simulink model "Demo_3D_FlexRoads_cs"  (R2014b)
settings: Solver=ode5  SolverMode=SingleTasking  StartTime=0.0  StopTime=107  FixedStep=1/200  RelTol=1e-3
PreLoadFcn:
  | mbxruntime.callbacks.PreLoadFcn(bdroot);
  | check_NUTS_defined;
  | 
  | assignin('base',['model_closed_' bdroot],false);
PostLoadFcn:
  | mbxruntime.callbacks.PostLoadFcn(bdroot);
InitFcn:
  | mbxruntime.callbacks.InitFcn(bdroot);
StartFcn:
  | mbxruntime.callbacks.StartFcn(bdroot);
StopFcn:
  | mbxruntime.callbacks.StopFcn(bdroot);
model workspace: external: MAT-File .\Demo_3D_FlexRoads_cs_hws.mat (data not in the file)
undefined symbols (not defined in the file or in its folder): InitImageOutputDir, warningInitialVelocity, x0
undefined symbols (not defined in the file): Demo_3D_FlexRoads_cs_51f4b8db1f5c5ce4, Demo_3D_FlexRoads_cs_6db096e0daa372af, Demo_3D_FlexRoads_cs_Audi_A8_1_Dynamics_Simple_3D_initialPitch, Demo_3D_FlexRoads_cs_Audi_A8_1_Dynamics_Simple_3D_initialRoll, Demo_3D_FlexRoads_cs_Audi_A8_1_Dynamics_Simple_3D_initialX, Demo_3D_FlexRoads_cs_Audi_A8_1_Dynamics_Simple_3D_initialY, Demo_3D_FlexRoads_cs_Audi_A8_1_Dynamics_Simple_3D_initialYaw, Demo_3D_FlexRoads_cs_Audi_A8_1_Dynamics_Simple_3D_initialZ, Demo_3D_FlexRoads_cs_Audi_A8_1_PreScan_Contact_Sensor_Pitch0, Demo_3D_FlexRoads_cs_Audi_A8_1_PreScan_Contact_Sensor_Roll0, Demo_3D_FlexRoads_cs_Audi_A8_1_PreScan_Contact_Sensor_x0, Demo_3D_FlexRoads_cs_Audi_A8_1_PreScan_Contact_Sensor_y0, Demo_3D_FlexRoads_cs_Audi_A8_1_PreScan_Contact_Sensor_Yaw0, Demo_3D_FlexRoads_cs_Audi_A8_1_PreScan_Contact_Sensor_z0, Demo_3D_FlexRoads_cs_Ford_FocusWagon_1_Path_pathUniqueID, WheelL0, WheelL1, WheelR0, WheelR1
libraries: simulink x34, simulink_extras x10, PreScanSimulinkLibrary x7
(part 5 of 6)

== system Demo_3D_FlexRoads_cs/Audi_A8_1/PreScan_Contact_Sensor/Wheels Local to World/conv_TransWheelFR ==
  transISO [m] : Inport
  Gain1 : Gain  Gain=Gain_xISO
  Gain2 : Gain  Gain=Gain_yISO
  Gain3 : Gain  Gain=Gain_zISO
  Mux2 : Mux  Inputs=3
  Sum : Sum  Inputs=|++
  pos_ini_Visu : Subsystem
  transISO2Visu : Subsystem
  transVisu [m] : Outport
  wires:
  Gain3/1 -> Mux2/3
  Gain2/1 -> Mux2/2
  Gain1/1 -> Mux2/1
  Sum/1 -> transVisu [m]/1
  pos_ini_Visu/1(pos_ini_Visu) -> Sum/2
  Mux2/1 -> Sum/1
  transISO [m]/1 -> transISO2Visu/1(transISO)
  transISO2Visu/1(trans_x_Visu) -> Gain1/1
  transISO2Visu/2(trans_y_Visu) -> Gain2/1
  transISO2Visu/3(trans_z_Visu) -> Gain3/1

== system Demo_3D_FlexRoads_cs/Audi_A8_1/PreScan_Contact_Sensor/Wheels Local to World/conv_TransWheelRL ==
  transISO [m] : Inport
  Gain1 : Gain  Gain=Gain_xISO
  Gain2 : Gain  Gain=Gain_yISO
  Gain3 : Gain  Gain=Gain_zISO
  Mux2 : Mux  Inputs=3
  Sum : Sum  Inputs=|++
  pos_ini_Visu : Subsystem
  transISO2Visu : Subsystem
  transVisu [m] : Outport
  wires:
  Gain3/1 -> Mux2/3
  Gain2/1 -> Mux2/2
  Gain1/1 -> Mux2/1
  Sum/1 -> transVisu [m]/1
  pos_ini_Visu/1(pos_ini_Visu) -> Sum/2
  Mux2/1 -> Sum/1
  transISO2Visu/3(trans_z_Visu) -> Gain3/1
  transISO2Visu/2(trans_y_Visu) -> Gain2/1
  transISO [m]/1 -> transISO2Visu/1(transISO)
  transISO2Visu/1(trans_x_Visu) -> Gain1/1

== system Demo_3D_FlexRoads_cs/Audi_A8_1/PreScan_Contact_Sensor/Wheels Local to World/conv_TransWheelRR ==
  transISO [m] : Inport
  Gain1 : Gain  Gain=Gain_xISO
  Gain2 : Gain  Gain=Gain_yISO
  Gain3 : Gain  Gain=Gain_zISO
  Mux2 : Mux  Inputs=3
  Sum : Sum  Inputs=|++
  pos_ini_Visu : Subsystem
  transISO2Visu : Subsystem
  transVisu [m] : Outport
  wires:
  Gain3/1 -> Mux2/3
  Gain2/1 -> Mux2/2
  Gain1/1 -> Mux2/1
  Sum/1 -> transVisu [m]/1
  pos_ini_Visu/1(pos_ini_Visu) -> Sum/2
  Mux2/1 -> Sum/1
  transISO2Visu/3(trans_z_Visu) -> Gain3/1
  transISO2Visu/2(trans_y_Visu) -> Gain2/1
  transISO [m]/1 -> transISO2Visu/1(transISO)
  transISO2Visu/1(trans_x_Visu) -> Gain1/1

== system Demo_3D_FlexRoads_cs/Audi_A8_1/SELF_Demux/compas converter/cart2compas ==
  Angle [deg] : Inport
  Constant : Constant  Value=90
  Constant1 : Constant  Value=360
  Gain : Gain  Gain=1/360
  Gain1 : Gain  Gain=360
  Gain2 : Gain  Gain=-1
  Rounding Function : Rounding
  Sum : Sum  Inputs=|-+
  Sum1 : Sum  Inputs=-+|
  Sum2 : Sum  Inputs=++|
  heading [deg] : Outport
  wires:
  Gain/1 -> Rounding Function/1
  Rounding Function/1 -> Gain1/1
  Gain1/1 -> Sum/1
  Angle [deg]/1 -> Sum1/2
  Sum/1 -> Gain2/1
  Sum1/1 -> Gain/1, Sum/2
  Constant/1 -> Sum1/1
  Gain2/1 -> Sum2/2
  Constant1/1 -> Sum2/1
  Sum2/1 -> heading [deg]/1

== system Demo_3D_FlexRoads_cs/Ford_FocusWagon_1/SELF_Demux/compas converter/cart2compas ==
  Angle [deg] : Inport
  Constant : Constant  Value=90
  Constant1 : Constant  Value=360
  Gain : Gain  Gain=1/360
  Gain1 : Gain  Gain=360
  Gain2 : Gain  Gain=-1
  Rounding Function : Rounding
  Sum : Sum  Inputs=|-+
  Sum1 : Sum  Inputs=-+|
  Sum2 : Sum  Inputs=++|
  heading [deg] : Outport
  wires:
  Gain/1 -> Rounding Function/1
  Rounding Function/1 -> Gain1/1
  Gain1/1 -> Sum/1
  Angle [deg]/1 -> Sum1/2
  Sum/1 -> Gain2/1
  Sum1/1 -> Gain/1, Sum/2
  Constant/1 -> Sum1/1
  Gain2/1 -> Sum2/2
  Constant1/1 -> Sum2/1
  Sum2/1 -> heading [deg]/1

== system Demo_3D_FlexRoads_cs/Audi_A8_1/Dynamics_Simple_3D/Chassis/Bicycle_model_[XYZ]/Fyi --> Fy // Mz ==
  DeltaWheel_[rad] : Inport
  Fy_f_[N] : Inport  Port=2
  Fy_r_[N] : Inport  Port=3
  Fy : Fcn  Expr=u(2)*cos(u(1)) + u(3)
  Mux1 : Mux  Inputs=3
  Mz : Fcn  Expr=u(2)*p.a*cos(u(1)) - u(3)*p.b
  Fy_[N] : Outport  InitialOutput=0
  Mz_[Nm] : Outport  Port=2  InitialOutput=0
  wires:
  DeltaWheel_[rad]/1 -> Mux1/1  "DeltaWheel_[rad]"
  Mz/1 -> Mz_[Nm]/1
  Fy/1 -> Fy_[N]/1
  Mux1/1 -> Mz/1, Fy/1
  Fy_f_[N]/1 -> Mux1/2
  Fy_r_[N]/1 -> Mux1/3

== system Demo_3D_FlexRoads_cs/Audi_A8_1/Dynamics_Simple_3D/Chassis/Bicycle_model_[XYZ]/RoadContact ==
  TyreInfo_in : Inport
  Penetration depth : Subsystem
  RoadGeometry : Subsystem
  depth_FL [m] : Outport
  depth_FR [m] : Outport  Port=2
  depth_RL [m] : Outport  Port=3
  depth_RR [m] : Outport  Port=4
  z : Outport  Port=5
  slope : Outport  Port=6
  banking : Outport  Port=7
  wires:
  Penetration depth/4(depth_RR [m]) -> depth_RR [m]/1
  Penetration depth/3(depth_RL [m]) -> depth_RL [m]/1
  Penetration depth/2(depth_FR [m]) -> depth_FR [m]/1
  Penetration depth/1(depth_FL [m]) -> depth_FL [m]/1
  TyreInfo_in/1 -> Penetration depth/1(TyreInfo_in), RoadGeometry/1(TyreInfo_in)
  RoadGeometry/1(z) -> z/1
  RoadGeometry/2(slope) -> slope/1
  RoadGeometry/3(banking) -> banking/1

== system Demo_3D_FlexRoads_cs/Audi_A8_1/Dynamics_Simple_3D/Chassis/Bicycle_model_[XYZ]/X_Motion ==
  DriveTorque_[Nm] : Inport
  BrakePressure_[bar] : Inport  Port=2
  v0_[ms-1] : Inport  Port=3
  slope_[rad] : Inport  Port=4
  vy_[ms-1] : Inport  Port=5
  dYaw_[rads-1] : Inport  Port=6
  Air&RoadResistance : Subsystem
  BrakeSystem : Subsystem
  Configurable Subsystem : Subsystem  BlockChoice=Discrete-Time Integrator  mask{ComputationMode=ComputationMode}
      mask prompts: ComputationMode "Computation mode:"
      mask init:
      | SetComputationMode(gcb,ComputationMode);
      settings: AttributesFormatString=%<BlockChoice>  OpenFcn=BringToFront(gcb);  MemberBlocks=Discrete-Time Integrator,Integrator
      settings: TemplateBlock=|
      | PreScanSimulinkLibrary/Configurable Subsystems/integral with reset and initial condition/Configurable
      | Subsystem
  Configurable Subsystem1 : Subsystem  BlockChoice=Discrete Torsional damping  mask{ComputationMode=ComputationMode}
      mask prompts: ComputationMode "Compuation mode:"
      mask init:
      | SetComputationMode(gcb,ComputationMode);
      settings: AttributesFormatString=%<BlockChoice>  OpenFcn=BringToFront(gcb);  MemberBlocks=Discrete Torsional damping,Torsional damping
      settings: TemplateBlock=|
      | PreScanSimulinkLibrary/Configurable Subsystems/TransferFunction
      | Torsional damping/Configurable
      | Subsystem
  Divide : Product  Inputs=**
  Gain : Gain  Gain=1/p.Rw
  Gain1 : Gain  Gain=p.Rw
  Max RPM and zero- velocity detection : Subsystem
  No contact rear wheels : Subsystem
  No contact wheels : Subsystem
  Slope Force : Subsystem
  Sum : Sum  Inputs=+-  SaturateOnIntegerOverflow=on  InputSameDT=on  OutDataTypeStr=Inherit: Same as first input
  Sum1 : Sum  SaturateOnIntegerOverflow=on  InputSameDT=on  OutDataTypeStr=Inherit: Same as first input
  Sum2 : Sum  Inputs=++-  SaturateOnIntegerOverflow=on  InputSameDT=on  OutDataTypeStr=Inherit: Same as first input
  inertia : Gain  Gain=1/p.m  SaturateOnIntegerOverflow=on  OutDataTypeStr=Inherit: Same as input  ParamDataTypeStr=Inherit: Same as input
  vx_[ms-1] : Outport
  ax_[ms-2] : Outport  Port=2
  wires:
  No contact rear wheels/1(ForceOut [N]) -> Sum/1
  Sum/1 -> Sum2/1  "sumForce_[N]"
  No contact wheels/1(ForceOut [N]) -> Sum2/3
  BrakeSystem/1(BrakeForce) -> No contact wheels/1(ForceIn [N])
  [slopeT] -> Max RPM and zero- velocity detection/3(Slope Torque)
  slope_[rad]/1 -> Slope Force/1(slope_[rad]), Air&RoadResistance/2(slope_[rad])
  Gain1/1 -> [slopeT]
  Slope Force/1(SlopeForce_[N]) -> Gain1/1, Sum2/2
  Gain/1 -> No contact rear wheels/1(ForceIn [N])
  Divide/1 -> Sum1/1
  dYaw_[rads-1]/1 -> Divide/2
  vy_[ms-1]/1 -> Divide/1
  BrakeSystem/2(BrakeTorqueAbs) -> [BT]
  [BT] -> Max RPM and zero- velocity detection/4(Brake Torque)
  [DT] -> Max RPM and zero- velocity detection/2(Drive Torque)
  v0_[ms-1]/1 -> Max RPM and zero- velocity detection/5(v0)
  Max RPM and zero- velocity detection/3(x0) -> Configurable Subsystem/3(In3)
  Max RPM and zero- velocity detection/2(vx_reset) -> Configurable Subsystem/2(In2)
  Max RPM and zero- velocity detection/1(ax_out) -> ax_[ms-2]/1, Configurable Subsystem/1(In1)  "ax [ms-2]"
  Configurable Subsystem1/1(Out1) -> Gain/1, [DT]
  Sum1/1 -> Max RPM and zero- velocity detection/1(ax)
  DriveTorque_[Nm]/1 -> Configurable Subsystem1/1(In1)  "DriveTorque_[Nm]"
  BrakePressure_[bar]/1 -> BrakeSystem/2(BrakePressure_[bar])  "BrakePressure_[bar]"
  Configurable Subsystem/1(Out1) -> Max RPM and zero- velocity detection/6(vx), BrakeSystem/1(vx_[ms-1]), Air&RoadResistance/1(vx_[ms-1]), vx_[ms-1]/1  "vx_[ms-1]"
  Air&RoadResistance/1(Resistance_Force) -> Sum/2
  Sum2/1 -> inertia/1
  inertia/1 -> Sum1/2  "dw[rads-2]"

== system Demo_3D_FlexRoads_cs/Audi_A8_1/Dynamics_Simple_3D/Chassis/Bicycle_model_[XYZ]/Y & Yaw_Motion ==
  |vx|_[ms-1] : Inport
  Fy_[N] : Inport  Port=2
  Mz_[Nm] : Inport  Port=3
  Compare To Zero : simulink/Logic and Bit Operations/Compare To Zero  relop===  OutDataTypeStr=boolean  ZeroCross=off
  Configurable Subsystem : Subsystem  BlockChoice=Discrete-Time Integrator  mask{ComputationMode=ComputationMode}
      mask prompts: ComputationMode "Computation mode:"
      mask init:
      | SetComputationMode(gcb,ComputationMode);
      settings: AttributesFormatString=%<BlockChoice>  OpenFcn=BringToFront(gcb);  MemberBlocks=Discrete-Time Integrator,Integrator
      settings: TemplateBlock=|
      | PreScanSimulinkLibrary/Configurable Subsystems/integral with reset/Configurable
      | Subsystem
  Configurable Subsystem1 : Subsystem  BlockChoice=Discrete-Time Integrator  mask{ComputationMode=ComputationMode}
      mask prompts: ComputationMode "Computation mode:"
      mask init:
      | SetComputationMode(gcb,ComputationMode);
      settings: AttributesFormatString=%<BlockChoice>  OpenFcn=BringToFront(gcb);  MemberBlocks=Discrete-Time Integrator,Integrator
      settings: TemplateBlock=|
      | PreScanSimulinkLibrary/Configurable Subsystems/integral with reset/Configurable
      | Subsystem
  Configurable Subsystem2 : Subsystem  BlockChoice=Discrete-Time Integrator  mask{ComputationMode=ComputationMode}
      link override Discrete-Time Integrator: IntegratorMethod=Integration: Backward Euler
      mask prompts: ComputationMode "Computation mode:"
      mask init:
      | SetComputationMode(gcb,ComputationMode);
      settings: AttributesFormatString=%<BlockChoice>  OpenFcn=BringToFront(gcb);  MemberBlocks=Discrete-Time Integrator,Integrator
      settings: TemplateBlock=|
      | PreScanSimulinkLibrary/Configurable Subsystems/integral/Configurable
      | Subsystem1
  Fcn1 : Fcn  Expr=u(1)*u(3)
  Gain : Gain  Gain=1/p.m  SaturateOnIntegerOverflow=on  OutDataTypeStr=Inherit: Same as input  ParamDataTypeStr=Inherit: Same as input
  Gain1 : Gain  Gain=1/p.J_zz  SaturateOnIntegerOverflow=on  OutDataTypeStr=Inherit: Same as input  ParamDataTypeStr=Inherit: Same as input
  Sum1 : Sum  Inputs=-+  SaturateOnIntegerOverflow=on  InputSameDT=on  OutDataTypeStr=Inherit: Same as first input
  mux : Mux  Inputs=3
  |vx|_[ms-1]1 : Outport  InitialOutput=0
  vy_[ms-1] : Outport  Port=2  InitialOutput=0
  ay_[ms-2] : Outport  Port=3  InitialOutput=0
  dYawAngle_[rads-1] : Outport  Port=4  InitialOutput=0
  YawAngle_[rad] : Outport  Port=5  InitialOutput=0
  wires:
  Configurable Subsystem1/1(Out1) -> mux/3, dYawAngle_[rads-1]/1, Configurable Subsystem2/1(In1)  "dYawAngle_[rads-1]"
  Configurable Subsystem/1(Out1) -> mux/2, vy_[ms-1]/1  "vy_[ms-1]"
  |vx|_[ms-1]/1 -> mux/1, |vx|_[ms-1]1/1, Compare To Zero/1  "|vx|_[ms-1]"
  mux/1 -> Fcn1/1  "|vx|_[ms-1]_vy_[ms-1]_dYawAngle_[rads-1]"
  Fcn1/1 -> Sum1/1  "|vx|*dYawAngle_[ms-2]"
  Sum1/1 -> Configurable Subsystem/1(In1)  "dvy_[ms-2]"
  Fy_[N]/1 -> Gain/1  "Fy_[N]"
  Mz_[Nm]/1 -> Gain1/1  "Mz_[Nm]"
  Configurable Subsystem2/1(Out1) -> YawAngle_[rad]/1
  Compare To Zero/1 -> [reset]
  [reset] -> Configurable Subsystem1/2(In2)
  [reset] -> Configurable Subsystem/2(In2)
  Gain/1 -> ay_[ms-2]/1, Sum1/2  "ddy_[ms-2]"
  Gain1/1 -> Configurable Subsystem1/1(In1)  "ddYawAngle_[rads-2]"

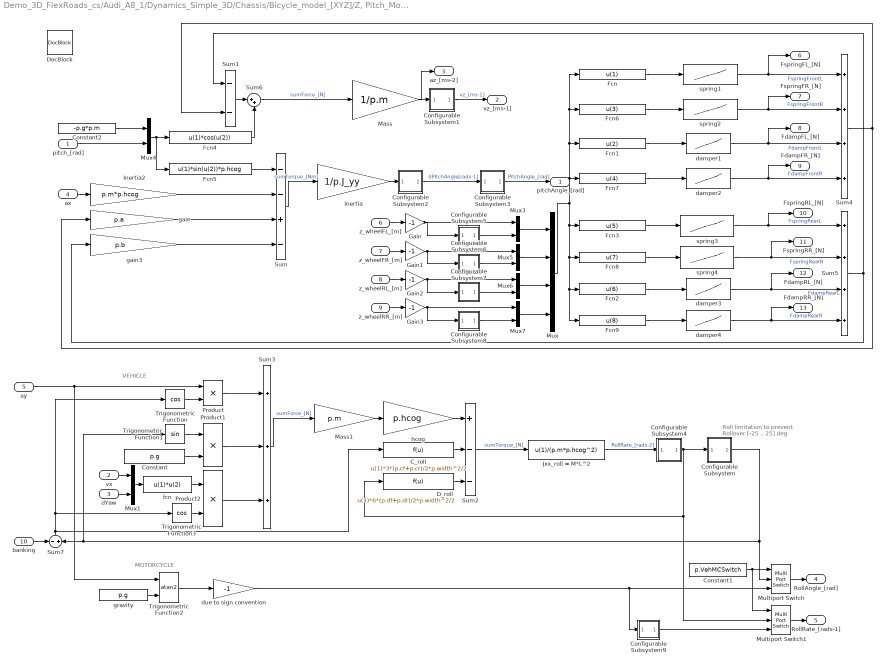
== system Demo_3D_FlexRoads_cs/Audi_A8_1/Dynamics_Simple_3D/Chassis/Bicycle_model_[XYZ]/Z, Pitch_Motion & Roll_Motion ==
  note: MOTORCYCLE
  note: Roll limitation
      | to prevent
      | Rollover
      | [-25 .. 25] deg
  note: VEHICLE
  pitch_[rad] : Inport
  vx : Inport  Port=2
  dYaw : Inport  Port=3
  ax : Inport  Port=4
  ay : Inport  Port=5
  z_wheelFL_[m] : Inport  Port=6
  z_wheelFR_[m] : Inport  Port=7
  z_wheelRL_[m] : Inport  Port=8
  z_wheelRR_[m] : Inport  Port=9
  banking : Inport  Port=10
  C_roll : Fcn  Expr=u(1)*3*(p.cf+p.cr)/2*p.width^2/2
  Configurable Subsystem : Subsystem  BlockChoice=Discrete-Time Integrator  mask{ComputationMode=ComputationMode}
      mask prompts: ComputationMode "Computation mode:"
      mask init:
      | SetComputationMode(gcb,ComputationMode);
      settings: AttributesFormatString=%<BlockChoice>  OpenFcn=BringToFront(gcb);  MemberBlocks=Discrete-Time Integrator,Integrator
      settings: TemplateBlock=|
      | PreScanSimulinkLibrary/Configurable Subsystems/integral with limits
      | for roll motion/Configurable
      | Subsystem
  Configurable Subsystem1 : Subsystem  BlockChoice=Discrete-Time Integrator  mask{ComputationMode=ComputationMode}
      mask prompts: ComputationMode "Computation mode:"
      mask init:
      | SetComputationMode(gcb,ComputationMode);
      settings: AttributesFormatString=%<BlockChoice>  OpenFcn=BringToFront(gcb);  MemberBlocks=Discrete-Time Integrator,Integrator
      settings: TemplateBlock=|
      | PreScanSimulinkLibrary/Configurable Subsystems/integral/Configurable
      | Subsystem1
  Configurable Subsystem2 : Subsystem  BlockChoice=Discrete-Time Integrator  mask{ComputationMode=ComputationMode}
      mask prompts: ComputationMode "Computation mode:"
      mask init:
      | SetComputationMode(gcb,ComputationMode);
      settings: AttributesFormatString=%<BlockChoice>  OpenFcn=BringToFront(gcb);  MemberBlocks=Discrete-Time Integrator,Integrator
      settings: TemplateBlock=|
      | PreScanSimulinkLibrary/Configurable Subsystems/integral/Configurable
      | Subsystem1
  Configurable Subsystem3 : Subsystem  BlockChoice=Discrete-Time Integrator  mask{ComputationMode=ComputationMode}
      mask prompts: ComputationMode "Computation mode:"
      mask init:
      | SetComputationMode(gcb,ComputationMode);
      settings: AttributesFormatString=%<BlockChoice>  OpenFcn=BringToFront(gcb);  MemberBlocks=Discrete-Time Integrator,Integrator
      settings: TemplateBlock=|
      | PreScanSimulinkLibrary/Configurable Subsystems/integral/Configurable
      | Subsystem1
  Configurable Subsystem4 : Subsystem  BlockChoice=Discrete-Time Integrator  mask{ComputationMode=ComputationMode}
      mask prompts: ComputationMode "Computation mode:"
      mask init:
      | SetComputationMode(gcb,ComputationMode);
      settings: AttributesFormatString=%<BlockChoice>  OpenFcn=BringToFront(gcb);  MemberBlocks=Discrete-Time Integrator,Integrator
      settings: TemplateBlock=|
      | PreScanSimulinkLibrary/Configurable Subsystems/integral/Configurable
      | Subsystem1
  Configurable Subsystem5 : Subsystem  BlockChoice=Discrete Derivative  mask{ComputationMode=ComputationMode}
      mask prompts: ComputationMode "Computation mode:"
      mask init:
      | SetComputationMode(gcb,ComputationMode);
      settings: AttributesFormatString=%<BlockChoice>  OpenFcn=BringToFront(gcb);  MemberBlocks=Derivative,Discrete Derivative
      settings: TemplateBlock=|
      | PreScanSimulinkLibrary/Configurable Subsystems/Derivative/Configurable
      | Subsystem
  Configurable Subsystem6 : Subsystem  BlockChoice=Discrete Derivative  mask{ComputationMode=ComputationMode}
      mask prompts: ComputationMode "Computation mode:"
      mask init:
      | SetComputationMode(gcb,ComputationMode);
      settings: AttributesFormatString=%<BlockChoice>  OpenFcn=BringToFront(gcb);  MemberBlocks=Derivative,Discrete Derivative
      settings: TemplateBlock=|
      | PreScanSimulinkLibrary/Configurable Subsystems/Derivative/Configurable
      | Subsystem
  Configurable Subsystem7 : Subsystem  BlockChoice=Discrete Derivative  mask{ComputationMode=ComputationMode}
      mask prompts: ComputationMode "Computation mode:"
      mask init:
      | SetComputationMode(gcb,ComputationMode);
      settings: AttributesFormatString=%<BlockChoice>  OpenFcn=BringToFront(gcb);  MemberBlocks=Derivative,Discrete Derivative
      settings: TemplateBlock=|
      | PreScanSimulinkLibrary/Configurable Subsystems/Derivative/Configurable
      | Subsystem
  Configurable Subsystem8 : Subsystem  BlockChoice=Discrete Derivative  mask{ComputationMode=ComputationMode}
      mask prompts: ComputationMode "Computation mode:"
      mask init:
      | SetComputationMode(gcb,ComputationMode);
      settings: AttributesFormatString=%<BlockChoice>  OpenFcn=BringToFront(gcb);  MemberBlocks=Derivative,Discrete Derivative
      settings: TemplateBlock=|
      | PreScanSimulinkLibrary/Configurable Subsystems/Derivative/Configurable
      | Subsystem
  Configurable Subsystem9 : Subsystem  BlockChoice=Discrete Derivative  mask{ComputationMode=ComputationMode}
      mask prompts: ComputationMode "Computation mode:"
      mask init:
      | SetComputationMode(gcb,ComputationMode);
      settings: AttributesFormatString=%<BlockChoice>  OpenFcn=BringToFront(gcb);  MemberBlocks=Derivative,Discrete Derivative
      settings: TemplateBlock=|
      | PreScanSimulinkLibrary/Configurable Subsystems/Derivative/Configurable
      | Subsystem
  Constant : Constant  Value=p.g
  Constant1 : Constant  Value=p.VehMCSwitch
  Constant2 : Constant  Value=-p.g*p.m
  D_roll : Fcn  Expr=u(1)*6*(p.df+p.dr)/2*p.width^2/2
  DocBlock : simulink/Model-Wide Utilities/DocBlock  DocumentType=Text
      content=|
      | This block determines the vertical, pitch and roll motions.
      |
      | The z motion is calculated by summing up all the forces that act in the
      | direction normal to the road:
      | - forces exerted by the suspensions (spring and dampers);
      | - vertical component of the force that is generated by the
      |   gravitational acceleration;
      | and then diving by the vehicle mass.
      |
      | The pitch motion is calculated by summing up all the torques that act
      | around the y-axis of the vehicle:
      | - forces exerted by the suspensions (spring and dampers);
      | - force generated by the longitudinal acceleration of the vehicle;
      | - longitudinal component of the force that is generated by the
      |   gravitational acceleration;
      | and then diving by the vehicle inertia moment around the pitch axis
      | (lugaroc: the position of the pitch axis has still to be formalized).
      |
      | The roll motion is calculated by summing up all the torques that act
      | around the x-axis of the vehicle (phi_a: absolute roll angle,
      | phi_r = phi_abs - beta: roll angle relative to the road):
      | - forces exerted by the suspensions (spring and dampers);
      | - component parallel to the vehicle y-axis of the forces generated by the
      |   lateral acceleration of the vehicle (cos(phi_r));
      | - component parallel to the vehicle y-axis of the force that is generated
      |   by the gravitational acceleration  (sin(phi_a));
      | and then diving by the vehicle inertia moment around the roll axis
      | (lugaroc: the inertia moment of the vehicle around the center of mass has
      | still to be included).
      |
      | For the calculation of the roll motion, the torques generated by the
      | suspension are equal to:
      |
      |   T_susproll = phi_r * K_roll + d(phi_r)/dt * C_roll
      |
      | where K_roll and C_roll are respectively the roll stiffness and damping.
      |
      | The calculation of the rolling velocity
      |
      |   d(phi_r)/dt = d(phi_a - beta)/dt = d(phi_a)/dt - d(beta)/dt
      |
      | requires the derivative of the road banking angle. This value is not
      | available and to avoid to apply the derivative of a discrete signal, the
      | equation is approximated as follows:
      |   d(phi_r)/dt = d(phi_a - beta)/dt =(approx) d(phi_a)/dt
      | thus d(beta)/dt is neglected.
  Fcn : Fcn  Expr=u(1)
  Fcn1 : Fcn  Expr=u(2)
  Fcn2 : Fcn  Expr=u(6)
  Fcn3 : Fcn  Expr=u(5)
  Fcn4 : Fcn  Expr=u(1)*cos(u(2))
  Fcn5 : Fcn  Expr=u(1)*sin(u(2))*p.hcog
  Fcn6 : Fcn  Expr=u(3)
  Fcn7 : Fcn  Expr=u(4)
  Fcn8 : Fcn  Expr=u(7)
  Fcn9 : Fcn  Expr=u(8)
  Gain{,1..3} (4 alike) : Gain  Gain=-1
  Inertia : Gain  Gain=1/p.J_yy  SaturateOnIntegerOverflow=on  OutDataTypeStr=Inherit: Same as input  ParamDataTypeStr=Inherit: Same as input
  Inertia2 : Gain  Gain=p.m*p.hcog  SaturateOnIntegerOverflow=on  OutDataTypeStr=Inherit: Same as input  ParamDataTypeStr=Inherit: Same as input
  Jxx_roll = M*L^2 : Fcn  Expr=u(1)/(p.m*p.hcog^2)
  Mass : Gain  Gain=1/p.m  SaturateOnIntegerOverflow=on  OutDataTypeStr=Inherit: Same as input  ParamDataTypeStr=Inherit: Same as input
  Mass1 : Gain  Gain=p.m  SaturateOnIntegerOverflow=on  OutDataTypeStr=Inherit: Same as input  ParamDataTypeStr=Inherit: Same as input
  Multiport Switch : MultiPortSwitch  Inputs=2
  Multiport Switch1 : MultiPortSwitch  Inputs=2
  Mux : Mux
  Mux{1,3..7} (6 alike) : Mux  Inputs=2
  Product : Product  RndMeth=Zero
  Product1 : Product  RndMeth=Zero
  Product2 : Product  RndMeth=Zero
  Sum : Sum  Inputs=--+-  SaturateOnIntegerOverflow=on  InputSameDT=on  OutDataTypeStr=Inherit: Same as first input
  Sum1 : Sum  Inputs=--  SaturateOnIntegerOverflow=on  InputSameDT=on  OutDataTypeStr=Inherit: Same as first input
  Sum2 : Sum  Inputs=+--  SaturateOnIntegerOverflow=on  InputSameDT=on  OutDataTypeStr=Inherit: Same as first input
  Sum3 : Sum  Inputs=+++  SaturateOnIntegerOverflow=on  InputSameDT=on  OutDataTypeStr=Inherit: Same as first input
  Sum4 : Sum  Inputs=++++  SaturateOnIntegerOverflow=on  InputSameDT=on  OutDataTypeStr=Inherit: Same as first input
  Sum5 : Sum  Inputs=++++  SaturateOnIntegerOverflow=on  InputSameDT=on  OutDataTypeStr=Inherit: Same as first input
  Sum6 : Sum  Inputs=|++
  Sum7 : Sum  Inputs=-|+
  Trigonometric Function : Trigonometry  Operator=cos
  Trigonometric Function1 : Trigonometry
  Trigonometric Function2 : Trigonometry  Operator=atan2
  Trigonometric Function3 : Trigonometry  Operator=cos
  damper1 : Lookup  InputValues=[p.suspDfrontVelDis]  Table=[p.suspDfrontFrc]
  damper2 : Lookup  InputValues=[p.suspDfrontVelDis]  Table=[p.suspDfrontFrc]
  damper3 : Lookup  InputValues=[p.suspDrearVelDis]  Table=[p.suspDrearFrc]
  damper4 : Lookup  InputValues=[p.suspDrearVelDis]  Table=[p.suspDrearFrc]
  due to sign convention : Gain  Gain=-1  SaturateOnIntegerOverflow=on  OutDataTypeStr=Inherit: Same as input  ParamDataTypeStr=Inherit: Same as input
  fcn : Fcn  Expr=u(1)*u(2)
  gain : Gain  Gain=p.a  SaturateOnIntegerOverflow=on  OutDataTypeStr=Inherit: Same as input  ParamDataTypeStr=Inherit: Same as input
  gain3 : Gain  Gain=p.b  SaturateOnIntegerOverflow=on  OutDataTypeStr=Inherit: Same as input  ParamDataTypeStr=Inherit: Same as input
  gravity : Constant  Value=p.g
  hcog : Gain  Gain=p.hcog  SaturateOnIntegerOverflow=on  OutDataTypeStr=Inherit: Same as input  ParamDataTypeStr=Inherit: Same as input
  spring1 : Lookup  InputValues=[p.suspKfrontDis]  Table=[p.suspKfrontFrc]
  spring2 : Lookup  InputValues=[p.suspKfrontDis]  Table=[p.suspKfrontFrc]
  spring3 : Lookup  InputValues=[p.suspKrearDis]  Table=[p.suspKrearFrc]
  spring4 : Lookup  InputValues=[p.suspKrearDis]  Table=[p.suspKrearFrc]
  pitchAngle_[rad] : Outport
  vz_[ms-1] : Outport  Port=2
  az_[ms-2] : Outport  Port=3
  RollAngle_[rad] : Outport  Port=4
  RollRate_[rads-1] : Outport  Port=5
  FspringFL_[N] : Outport  Port=6
  FspringFR_[N] : Outport  Port=7
  FdampFL_[N] : Outport  Port=8
  FdampFR_[N] : Outport  Port=9
  FspringRL_[N] : Outport  Port=10
  FspringRR_[N] : Outport  Port=11
  FdampRL_[N] : Outport  Port=12
  FdampRR_[N] : Outport  Port=13
  wires:
  Fcn2/1 -> damper3/1
  z_wheelRR_[m]/1 -> Gain3/1
  z_wheelRL_[m]/1 -> Gain2/1
  z_wheelFR_[m]/1 -> Gain1/1
  z_wheelFL_[m]/1 -> Gain/1
  Gain3/1 -> Mux7/1, Configurable Subsystem8/1(In1)
  Gain2/1 -> Mux6/1, Configurable Subsystem7/1(In1)
  Gain1/1 -> Mux5/1, Configurable Subsystem6/1(In1)
  Gain/1 -> Mux3/1, Configurable Subsystem5/1(In1)
  spring1/1 -> Sum4/1, FspringFL_[N]/1  "FspringFrontL"
  damper4/1 -> Sum5/4, FdampRR_[N]/1  "FdampRearR"
  spring4/1 -> Sum5/2, FspringRR_[N]/1  "FspringRearR"
  spring2/1 -> Sum4/2, FspringFR_[N]/1  "FspringFrontR"
  damper2/1 -> Sum4/4, FdampFR_[N]/1  "FdampFrontR"
  Fcn9/1 -> damper4/1
  Fcn8/1 -> spring4/1
  Fcn7/1 -> damper2/1
  Fcn6/1 -> spring2/1
  Mux7/1 -> Mux/4
  Mux6/1 -> Mux/3
  Mux5/1 -> Mux/2
  Mux3/1 -> Mux/1
  Configurable Subsystem8/1(Out1) -> Mux7/2
  Configurable Subsystem7/1(Out1) -> Mux6/2
  Configurable Subsystem6/1(Out1) -> Mux5/2
  Configurable Subsystem5/1(Out1) -> Mux3/2
  Configurable Subsystem9/1(Out1) -> Multiport Switch1/3
  Constant1/1 -> Multiport Switch1/1, Multiport Switch/1
  gravity/1 -> Trigonometric Function2/2
  Trigonometric Function2/1 -> due to sign convention/1
  due to sign convention/1 -> Multiport Switch/3, Configurable Subsystem9/1(In1)
  Product2/1 -> Sum3/3
  Trigonometric Function3/1 -> Product2/2
  fcn/1 -> Product2/1
  dYaw/1 -> Mux1/2
  vx/1 -> Mux1/1
  Mux1/1 -> fcn/1
  Multiport Switch1/1 -> RollRate_[rads-1]/1
  Multiport Switch/1 -> RollAngle_[rad]/1
  D_roll/1 -> Sum2/3
  C_roll/1 -> Sum2/2
  hcog/1 -> Sum2/1
  Mass1/1 -> hcog/1
  Sum3/1 -> Mass1/1  "sumForce_[N]"
  Product1/1 -> Sum3/2
  Product/1 -> Sum3/1
  Constant/1 -> Product1/2
  Trigonometric Function1/1 -> Product1/1
  ay/1 -> Trigonometric Function2/1, Product/1
  Trigonometric Function/1 -> Product/2
  Configurable Subsystem/1(Out1) -> Multiport Switch/2, Sum7/2, Trigonometric Function1/1
  Configurable Subsystem4/1(Out1) -> Multiport Switch1/2, D_roll/1, Configurable Subsystem/1(In1)
  Jxx_roll = M*L^2/1 -> Configurable Subsystem4/1(In1)  "RollRate_[rads-2]"
  Sum2/1 -> Jxx_roll = M*L^2/1  "sumTorque_[N]"
  gain3/1 -> Sum/4
  gain/1 -> Sum/3
  Inertia2/1 -> Sum/2
  Fcn5/1 -> Sum/1
  Configurable Subsystem3/1(Out1) -> pitchAngle_[rad]/1  "PitchAngle_[rad]"
  Sum1/1 -> Sum6/1
  Sum/1 -> Inertia/1  "sumTorque_[Nm]"
  damper3/1 -> Sum5/3, FdampRL_[N]/1  "FdampRearL"
  Fcn4/1 -> Sum6/2
  Constant2/1 -> Mux4/1
  pitch_[rad]/1 -> Mux4/2
  Mux4/1 -> Fcn5/1, Fcn4/1
  Fcn/1 -> spring1/1
  Fcn3/1 -> spring3/1
  Fcn1/1 -> damper1/1
  Sum6/1 -> Mass/1  "sumForce_[N]"
  Mass/1 -> az_[ms-2]/1, Configurable Subsystem1/1(In1)
  Mux/1 -> Fcn3/1, Fcn8/1, Fcn9/1, Fcn2/1, Fcn7/1, Fcn6/1, Fcn/1, Fcn1/1
  Sum5/1 -> Sum1/1, gain3/1
  Sum4/1 -> Sum1/2, gain/1
  spring3/1 -> FspringRL_[N]/1, Sum5/1  "FspringRearL"
  damper1/1 -> Sum4/3, FdampFL_[N]/1  "FdampFrontL"
  ax/1 -> Inertia2/1
  Configurable Subsystem1/1(Out1) -> vz_[ms-1]/1  "vz_[ms-1]"
  Configurable Subsystem2/1(Out1) -> Configurable Subsystem3/1(In1)  "dPitchAngle[rads-1]"
  Inertia/1 -> Configurable Subsystem2/1(In1)
  banking/1 -> Sum7/1
  Sum7/1 -> C_roll/1, Trigonometric Function/1, Trigonometric Function3/1

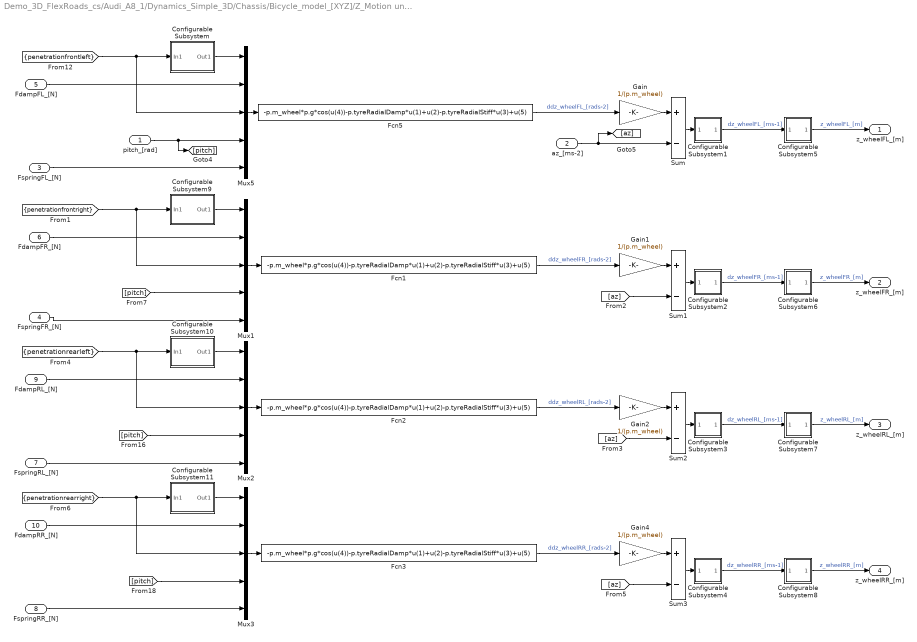
== system Demo_3D_FlexRoads_cs/Audi_A8_1/Dynamics_Simple_3D/Chassis/Bicycle_model_[XYZ]/Z_Motion unsprung mass ==
  pitch_[rad] : Inport
  az_[ms-2] : Inport  Port=2
  FspringFL_[N] : Inport  Port=3
  FspringFR_[N] : Inport  Port=4
  FdampFL_[N] : Inport  Port=5
  FdampFR_[N] : Inport  Port=6
  FspringRL_[N] : Inport  Port=7
  FspringRR_[N] : Inport  Port=8
  FdampRL_[N] : Inport  Port=9
  FdampRR_[N] : Inport  Port=10
  Configurable Subsystem : Subsystem  BlockChoice=Derivative  mask{ComputationMode=ComputationMode}
      mask prompts: ComputationMode "Computation mode:"
      mask init:
      | SetComputationMode(gcb,ComputationMode);
      settings: AttributesFormatString=%<BlockChoice>  OpenFcn=BringToFront(gcb);  MemberBlocks=Derivative,Discrete Derivative
      settings: TemplateBlock=|
      | PreScanSimulinkLibrary/Configurable Subsystems/Derivative/Configurable
      | Subsystem
  Configurable Subsystem1 : Subsystem  BlockChoice=Integrator  mask{ComputationMode=ComputationMode}
      mask prompts: ComputationMode "Computation mode:"
      mask init:
      | SetComputationMode(gcb,ComputationMode);
      settings: AttributesFormatString=%<BlockChoice>  OpenFcn=BringToFront(gcb);  MemberBlocks=Discrete-Time Integrator,Integrator
      settings: TemplateBlock=|
      | PreScanSimulinkLibrary/Configurable Subsystems/integral Backward Euler/Configurable
      | Subsystem1
  Configurable Subsystem10 : Subsystem  BlockChoice=Derivative  mask{ComputationMode=ComputationMode}
      mask prompts: ComputationMode "Computation mode:"
      mask init:
      | SetComputationMode(gcb,ComputationMode);
      settings: AttributesFormatString=%<BlockChoice>  OpenFcn=BringToFront(gcb);  MemberBlocks=Derivative,Discrete Derivative
      settings: TemplateBlock=|
      | PreScanSimulinkLibrary/Configurable Subsystems/Derivative/Configurable
      | Subsystem
  Configurable Subsystem11 : Subsystem  BlockChoice=Derivative  mask{ComputationMode=ComputationMode}
      mask prompts: ComputationMode "Computation mode:"
      mask init:
      | SetComputationMode(gcb,ComputationMode);
      settings: AttributesFormatString=%<BlockChoice>  OpenFcn=BringToFront(gcb);  MemberBlocks=Derivative,Discrete Derivative
      settings: TemplateBlock=|
      | PreScanSimulinkLibrary/Configurable Subsystems/Derivative/Configurable
      | Subsystem
  Configurable Subsystem2 : Subsystem  BlockChoice=Integrator  mask{ComputationMode=ComputationMode}
      mask prompts: ComputationMode "Computation mode:"
      mask init:
      | SetComputationMode(gcb,ComputationMode);
      settings: AttributesFormatString=%<BlockChoice>  OpenFcn=BringToFront(gcb);  MemberBlocks=Discrete-Time Integrator,Integrator
      settings: TemplateBlock=|
      | PreScanSimulinkLibrary/Configurable Subsystems/integral Backward Euler/Configurable
      | Subsystem1
  Configurable Subsystem3 : Subsystem  BlockChoice=Integrator  mask{ComputationMode=ComputationMode}
      mask prompts: ComputationMode "Computation mode:"
      mask init:
      | SetComputationMode(gcb,ComputationMode);
      settings: AttributesFormatString=%<BlockChoice>  OpenFcn=BringToFront(gcb);  MemberBlocks=Discrete-Time Integrator,Integrator
      settings: TemplateBlock=|
      | PreScanSimulinkLibrary/Configurable Subsystems/integral Backward Euler/Configurable
      | Subsystem1
  Configurable Subsystem4 : Subsystem  BlockChoice=Integrator  mask{ComputationMode=ComputationMode}
      mask prompts: ComputationMode "Computation mode:"
      mask init:
      | SetComputationMode(gcb,ComputationMode);
      settings: AttributesFormatString=%<BlockChoice>  OpenFcn=BringToFront(gcb);  MemberBlocks=Discrete-Time Integrator,Integrator
      settings: TemplateBlock=|
      | PreScanSimulinkLibrary/Configurable Subsystems/integral Backward Euler/Configurable
      | Subsystem1
  Configurable Subsystem5 : Subsystem  BlockChoice=Integrator  mask{ComputationMode=ComputationMode}
      mask prompts: ComputationMode "Computation mode:"
      mask init:
      | SetComputationMode(gcb,ComputationMode);
      settings: AttributesFormatString=%<BlockChoice>  OpenFcn=BringToFront(gcb);  MemberBlocks=Discrete-Time Integrator,Integrator
      settings: TemplateBlock=|
      | PreScanSimulinkLibrary/Configurable Subsystems/integral/Configurable
      | Subsystem1
  Configurable Subsystem6 : Subsystem  BlockChoice=Integrator  mask{ComputationMode=ComputationMode}
      mask prompts: ComputationMode "Computation mode:"
      mask init:
      | SetComputationMode(gcb,ComputationMode);
      settings: AttributesFormatString=%<BlockChoice>  OpenFcn=BringToFront(gcb);  MemberBlocks=Discrete-Time Integrator,Integrator
      settings: TemplateBlock=|
      | PreScanSimulinkLibrary/Configurable Subsystems/integral/Configurable
      | Subsystem1
  Configurable Subsystem7 : Subsystem  BlockChoice=Integrator  mask{ComputationMode=ComputationMode}
      mask prompts: ComputationMode "Computation mode:"
      mask init:
      | SetComputationMode(gcb,ComputationMode);
      settings: AttributesFormatString=%<BlockChoice>  OpenFcn=BringToFront(gcb);  MemberBlocks=Discrete-Time Integrator,Integrator
      settings: TemplateBlock=|
      | PreScanSimulinkLibrary/Configurable Subsystems/integral/Configurable
      | Subsystem1
  Configurable Subsystem8 : Subsystem  BlockChoice=Integrator  mask{ComputationMode=ComputationMode}
      mask prompts: ComputationMode "Computation mode:"
      mask init:
      | SetComputationMode(gcb,ComputationMode);
      settings: AttributesFormatString=%<BlockChoice>  OpenFcn=BringToFront(gcb);  MemberBlocks=Discrete-Time Integrator,Integrator
      settings: TemplateBlock=|
      | PreScanSimulinkLibrary/Configurable Subsystems/integral/Configurable
      | Subsystem1
  Configurable Subsystem9 : Subsystem  BlockChoice=Derivative  mask{ComputationMode=ComputationMode}
      mask prompts: ComputationMode "Computation mode:"
      mask init:
      | SetComputationMode(gcb,ComputationMode);
      settings: AttributesFormatString=%<BlockChoice>  OpenFcn=BringToFront(gcb);  MemberBlocks=Derivative,Discrete Derivative
      settings: TemplateBlock=|
      | PreScanSimulinkLibrary/Configurable Subsystems/Derivative/Configurable
      | Subsystem
  Fcn{1..3,5} (4 alike) : Fcn  Expr=-p.m_wheel*p.g*cos(u(4))-p.tyreRadialDamp*u(1)+u(2)-p.tyreRadialStiff*u(3)+u(5)
  Gain{,1..2,4} (4 alike) : Gain  Gain=1/(p.m_wheel)
  Mux{1..3,5} (4 alike) : Mux  Inputs=5
  Sum{,1..3} (4 alike) : Sum  Inputs=+-
  z_wheelFL_[m] : Outport
  z_wheelFR_[m] : Outport  Port=2
  z_wheelRL_[m] : Outport  Port=3
  z_wheelRR_[m] : Outport  Port=4
  wires:
  Configurable Subsystem7/1(Out1) -> z_wheelRL_[m]/1  "z_wheelRL_[m]"
  [pitch] -> Mux1/4
  FdampFR_[N]/1 -> Mux1/2
  [pitch] -> Mux3/4
  [pitch] -> Mux2/4
  pitch_[rad]/1 -> Mux5/4, [pitch]
  [az] -> Sum3/2
  [az] -> Sum2/2
  [az] -> Sum1/2
  az_[ms-2]/1 -> [az], Sum/2
  FdampRR_[N]/1 -> Mux3/2
  FdampRL_[N]/1 -> Mux2/2
  FdampFL_[N]/1 -> Mux5/2
  FspringRR_[N]/1 -> Mux3/5
  FspringRL_[N]/1 -> Mux2/5
  FspringFR_[N]/1 -> Mux1/5
  FspringFL_[N]/1 -> Mux5/5
  Sum3/1 -> Configurable Subsystem4/1(In1)
  Gain4/1 -> Sum3/1
  Sum2/1 -> Configurable Subsystem3/1(In1)
  Gain2/1 -> Sum2/1
  Sum1/1 -> Configurable Subsystem2/1(In1)
  Gain1/1 -> Sum1/1
  Sum/1 -> Configurable Subsystem1/1(In1)
  Gain/1 -> Sum/1
  [penetrationrearleft] -> Mux2/3, Configurable Subsystem10/1(In1)
  [penetrationrearright] -> Mux3/3, Configurable Subsystem11/1(In1)
  Mux3/1 -> Fcn3/1
  Configurable Subsystem11/1(Out1) -> Mux3/1
  Configurable Subsystem8/1(Out1) -> z_wheelRR_[m]/1  "z_wheelRR_[m]"
  Configurable Subsystem4/1(Out1) -> Configurable Subsystem8/1(In1)  "dz_wheelRR_[ms-1]"
  Fcn3/1 -> Gain4/1  "ddz_wheelRR_[rads-2]"
  Mux2/1 -> Fcn2/1
  Configurable Subsystem10/1(Out1) -> Mux2/1
  Configurable Subsystem3/1(Out1) -> Configurable Subsystem7/1(In1)  "dz_wheelRL_[ms-1]"
  Fcn2/1 -> Gain2/1  "ddz_wheelRL_[rads-2]"
  [penetrationfrontright] -> Mux1/3, Configurable Subsystem9/1(In1)
  Mux1/1 -> Fcn1/1
  Configurable Subsystem9/1(Out1) -> Mux1/1
  Configurable Subsystem6/1(Out1) -> z_wheelFR_[m]/1  "z_wheelFR_[m]"
  Configurable Subsystem2/1(Out1) -> Configurable Subsystem6/1(In1)  "dz_wheelFR_[ms-1]"
  Fcn1/1 -> Gain1/1  "ddz_wheelFR_[rads-2]"
  [penetrationfrontleft] -> Mux5/3, Configurable Subsystem/1(In1)
  Mux5/1 -> Fcn5/1
  Configurable Subsystem/1(Out1) -> Mux5/1
  Configurable Subsystem5/1(Out1) -> z_wheelFL_[m]/1  "z_wheelFL_[m]"
  Configurable Subsystem1/1(Out1) -> Configurable Subsystem5/1(In1)  "dz_wheelFL_[ms-1]"
  Fcn5/1 -> Gain/1  "ddz_wheelFL_[rads-2]"

== system Demo_3D_FlexRoads_cs/Audi_A8_1/Dynamics_Simple_3D/Chassis/FrontTyre/AlphaFront ==
  In : Inport
  Abs : Abs
  Compare To Constant : simulink/Logic and Bit Operations/Compare To Constant  relop=>  const=0  OutDataTypeStr=uint8  ZeroCross=off
  Enabled Subsystem : Subsystem  TreatAsAtomicUnit=on
  Selector : Selector
  Alpha : Outport
  wires:
  Selector/1 -> Abs/1
  Compare To Constant/1 -> Enabled Subsystem/Enable
  Enabled Subsystem/1(Alpha) -> Alpha/1
  In/1 -> Enabled Subsystem/1(In), Selector/1
  Abs/1 -> Compare To Constant/1

== system Demo_3D_FlexRoads_cs/Audi_A8_1/Dynamics_Simple_3D/Chassis/FrontTyre/Configurable Subsystem ==
  In1 : Inport
  In2 : Inport  Port=2
  Discrete-Time Integrator : DiscreteIntegrator  ExternalReset=level  SampleTime=TimeStep  LimitOutput=on  UpperSaturationLimit=1  LowerSaturationLimit=-1
  Out1 : Outport
  wires:
  In1/1 -> Discrete-Time Integrator/1
  In2/1 -> Discrete-Time Integrator/2
  Discrete-Time Integrator/1 -> Out1/1

== system Demo_3D_FlexRoads_cs/Audi_A8_1/Dynamics_Simple_3D/Chassis/FrontTyre/Configurable Subsystem1 ==
  In1 : Inport
  In2 : Inport  Port=2
  Discrete-Time Integrator : DiscreteIntegrator  ExternalReset=level  SampleTime=TimeStep
  Out1 : Outport
  wires:
  In1/1 -> Discrete-Time Integrator/1
  In2/1 -> Discrete-Time Integrator/2
  Discrete-Time Integrator/1 -> Out1/1

== system Demo_3D_FlexRoads_cs/Audi_A8_1/Dynamics_Simple_3D/Chassis/RearTyre/AlphaRear ==
  In : Inport
  Abs : Abs
  Compare To Constant : simulink/Logic and Bit Operations/Compare To Constant  relop=>  const=0  OutDataTypeStr=uint8  ZeroCross=off
  Enabled Subsystem : Subsystem  TreatAsAtomicUnit=on
  Selector : Selector
  Alpha : Outport
  wires:
  Selector/1 -> Abs/1
  Compare To Constant/1 -> Enabled Subsystem/Enable
  Enabled Subsystem/1(Alpha) -> Alpha/1
  In/1 -> Enabled Subsystem/1(In), Selector/1
  Abs/1 -> Compare To Constant/1

== system Demo_3D_FlexRoads_cs/Audi_A8_1/Dynamics_Simple_3D/Chassis/RearTyre/Configurable Subsystem ==
  In1 : Inport
  In2 : Inport  Port=2
  Discrete-Time Integrator : DiscreteIntegrator  ExternalReset=level  SampleTime=TimeStep  LimitOutput=on  UpperSaturationLimit=1  LowerSaturationLimit=-1
  Out1 : Outport
  wires:
  In1/1 -> Discrete-Time Integrator/1
  In2/1 -> Discrete-Time Integrator/2
  Discrete-Time Integrator/1 -> Out1/1

== system Demo_3D_FlexRoads_cs/Audi_A8_1/Dynamics_Simple_3D/Chassis/RearTyre/Configurable Subsystem1 ==
  In1 : Inport
  In2 : Inport  Port=2
  Discrete-Time Integrator : DiscreteIntegrator  ExternalReset=level  SampleTime=TimeStep
  Out1 : Outport
  wires:
  In1/1 -> Discrete-Time Integrator/1
  In2/1 -> Discrete-Time Integrator/2
  Discrete-Time Integrator/1 -> Out1/1

== system Demo_3D_FlexRoads_cs/Audi_A8_1/Dynamics_Simple_3D/ShiftLogic/Detect Increase/If V0 higher of the from 2->3 shifting velocity ==
  In1 : Inport
  Action Port : ActionPort  PropagateVarSize=During execution
  Out1 : Outport
  wires:
  In1/1 -> Out1/1

== system Demo_3D_FlexRoads_cs/Audi_A8_1/Dynamics_Simple_3D/ShiftLogic/Detect Increase/Other ==
  In1 : Inport
  Action Port : ActionPort  PropagateVarSize=During execution
  Data Type Conversion : DataTypeConversion  OutDataTypeStr=double
  Detect Increase : simulink/Logic and Bit Operations/Detect Increase  vinit=0.0  InputProcessing=Inherited  OutDataTypeStr=uint8
  Out1 : Outport
  wires:
  Data Type Conversion/1 -> Out1/1
  Detect Increase/1 -> Data Type Conversion/1
  In1/1 -> Detect Increase/1

== system Demo_3D_FlexRoads_cs/Audi_A8_1/Dynamics_Simple_3D/Transmission/Transmission_Ratio/If Action Neutral ==
  In1 : Inport
  Action Port : ActionPort  InitializeStates=reset  PropagateVarSize=During execution
  Out1 : Outport
  wires:
  In1/1 -> Out1/1

== system Demo_3D_FlexRoads_cs/Audi_A8_1/Dynamics_Simple_3D/Transmission/Transmission_Ratio/If Action Normal ==
  In1 : Inport
  Action Port : ActionPort  InitializeStates=reset  PropagateVarSize=During execution
  Out1 : Outport
  wires:
  In1/1 -> Out1/1

== system Demo_3D_FlexRoads_cs/Audi_A8_1/Dynamics_Simple_3D/Transmission/Transmission_Ratio/If Action Reverse ==
  In1 : Inport
  Action Port : ActionPort  InitializeStates=reset  PropagateVarSize=During execution
  Reverse : Gain  Gain=-1
  Out1 : Outport
  wires:
  In1/1 -> Reverse/1
  Reverse/1 -> Out1/1

== system Demo_3D_FlexRoads_cs/Audi_A8_1/PathFollower_Preview_1/LateralController/SteeringWheelAngle/FirstOrderDynamics ==
  In : Inport
  TimeConstant[s] : Inport  Port=2
  Reset : Inport  Port=3
  x0 : Inport  Port=4
  1|TimeConstant : Product  Inputs=*/  SaturateOnIntegerOverflow=on  InputSameDT=on  OutDataTypeStr=Inherit: Same as first input
  Discrete-Time Integrator : DiscreteIntegrator  ExternalReset=rising  InitialConditionSource=external  InitialCondition=x0  SampleTime=CSSampleTime
  IC : InitialCondition  Value=0
  Saturation : Saturate  UpperLimit=1e300  LowerLimit=0.001
  Sum : Sum  Inputs=-+|  SaturateOnIntegerOverflow=on  InputSameDT=on  OutDataTypeStr=Inherit: Same as first input
  Out : Outport
  wires:
  IC/1 -> Discrete-Time Integrator/3
  In/1 -> Sum/2
  x0/1 -> IC/1
  Reset/1 -> Discrete-Time Integrator/2
  1|TimeConstant/1 -> Discrete-Time Integrator/1
  Sum/1 -> 1|TimeConstant/1
  Saturation/1 -> 1|TimeConstant/2
  TimeConstant[s]/1 -> Saturation/1
  Discrete-Time Integrator/1 -> Out/1, Sum/1

== system Demo_3D_FlexRoads_cs/Audi_A8_1/PathFollower_Preview_1/LateralController/SteeringWheelAngle/Sat_Total ==
  In : Inport
  Sat_Limit : Inport  Port=2
  Gain1 : Gain  Gain=-1  SaturateOnIntegerOverflow=on  OutDataTypeStr=Inherit: Same as input  ParamDataTypeStr=Inherit: Same as input
  RelOp_UL : RelationalOperator
  RelOp_UL1 : RelationalOperator  Operator=<=
  Sum : Sum  Inputs=++|  SaturateOnIntegerOverflow=on
  Switch : Switch  Threshold=0.5  SaturateOnIntegerOverflow=on
  Switch1 : Switch  Threshold=0.5  SaturateOnIntegerOverflow=on
  Sat_Total : Outport
  Sat_Info : Outport  Port=2
  wires:
  Sat_Limit/1 -> Gain1/1, Switch/1, RelOp_UL/2
  RelOp_UL/1 -> Switch/2, Sum/2
  Switch/1 -> RelOp_UL1/1, Switch1/3
  Gain1/1 -> RelOp_UL1/2, Switch1/1
  RelOp_UL1/1 -> Switch1/2, Sum/1
  In/1 -> Switch/3, RelOp_UL/1
  Switch1/1 -> Sat_Total/1
  Sum/1 -> Sat_Info/1

== system Demo_3D_FlexRoads_cs/Audi_A8_1/PathFollower_Preview_1/LongitudinalController/If Desired Velocity ~= 0/PID_AWU ==
  e : Inport
  Derivative Gain : Gain  Gain=D  SaturateOnIntegerOverflow=on  OutDataTypeStr=Inherit: Same as input  ParamDataTypeStr=Inherit: Same as input
  Discrete-Time Integrator : DiscreteIntegrator  gainval=1  SampleTime=CSSampleTime  UpperSaturationLimit=100  LowerSaturationLimit=-100
  Filter : DiscreteIntegrator  gainval=1  SampleTime=CSSampleTime
  Integral Gain : Gain  Gain=I  SaturateOnIntegerOverflow=on  OutDataTypeStr=Inherit: Same as input  ParamDataTypeStr=Inherit: Same as input
  Integral Gain1 : Gain  Gain=LongCtrl_AWU  SaturateOnIntegerOverflow=on  OutDataTypeStr=Inherit: Same as input  ParamDataTypeStr=Inherit: Same as input
  Proportional Gain : Gain  Gain=P  SaturateOnIntegerOverflow=on  OutDataTypeStr=Inherit: Same as input  ParamDataTypeStr=Inherit: Same as input
  Saturation : Saturate  UpperLimit=100  LowerLimit=-100
  Sum : Sum  Inputs=+++  SaturateOnIntegerOverflow=on  InputSameDT=on  OutDataTypeStr=Inherit: Same as first input
  Sum1 : Sum  Inputs=|+-  SaturateOnIntegerOverflow=on  InputSameDT=on  OutDataTypeStr=Inherit: Same as first input
  Sum2 : Sum  Inputs=|++  SaturateOnIntegerOverflow=on  InputSameDT=on  OutDataTypeStr=Inherit: Same as first input
  Sum3 : Sum  Inputs=-+|  SaturateOnIntegerOverflow=on  InputSameDT=on  OutDataTypeStr=Inherit: Same as first input
  u : Outport  InitialOutput=0
  wires:
  Integral Gain1/1 -> Sum2/2
  Sum3/1 -> Integral Gain1/1
  Saturation/1 -> Sum3/2, u/1
  Sum2/1 -> Discrete-Time Integrator/1
  Sum1/1 -> Sum/3, Filter/1
  Filter/1 -> Sum1/2
  Derivative Gain/1 -> Sum1/1
  Sum/1 -> Sum3/1, Saturation/1
  e/1 -> Integral Gain/1, Proportional Gain/1, Derivative Gain/1
  Discrete-Time Integrator/1 -> Sum/2
  Proportional Gain/1 -> Sum/1
  Integral Gain/1 -> Sum2/1

== system Demo_3D_FlexRoads_cs/Audi_A8_1/PreScan_Contact_Sensor/Vehicle Local to World/state2FullState/Transformation_BODY2GLOBAL1 ==
  POSvector_BODY_[m] : Inport
  angles_BODYwrtGLOB_[rad] : Inport  Port=2
  Dot Product : DotProduct  InputSameDT=on  OutDataTypeStr=Inherit: Inherit via internal rule
  Dot Product1 : DotProduct  InputSameDT=on  OutDataTypeStr=Inherit: Inherit via internal rule
  Dot Product2 : DotProduct  InputSameDT=on  OutDataTypeStr=Inherit: Inherit via internal rule
  Fcn10 : Fcn  Expr=cos(u(1))*sin(u(2))*sin(u(3))-sin(u(1))*cos(u(3))
  Fcn11 : Fcn  Expr=cos(u(1))*sin(u(2))*cos(u(3))+sin(u(1))*sin(u(3))
  Fcn12 : Fcn  Expr=sin(u(1))*cos(u(2))
  Fcn13 : Fcn  Expr=sin(u(1))*sin(u(2))*sin(u(3))+cos(u(1))*cos(u(3))
  Fcn14 : Fcn  Expr=sin(u(1))*sin(u(2))*cos(u(3))-cos(u(1))*sin(u(3))
  Fcn15 : Fcn  Expr=-sin(u(2))
  Fcn16 : Fcn  Expr=cos(u(2))*sin(u(3))
  Fcn17 : Fcn  Expr=cos(u(2))*cos(u(3))
  Fcn9 : Fcn  Expr=cos(u(1))*cos(u(2))
  Mux1 : Mux  Inputs=9
  Mux3 : Mux  Inputs=3
  Selector : Selector  InputPortWidth=9  Indices=[1 2 3]
  Selector1 : Selector  InputPortWidth=9  Indices=[4 5 6]
  Selector2 : Selector  InputPortWidth=9  Indices=[7 8 9]
  rot_xyz 2 rot_zyx : Selector  InputPortWidth=3  Indices=[3 2 1]
  POSvector_GLOBAL_[m] : Outport
  wires:
  Fcn9/1 -> Mux1/1
  Fcn10/1 -> Mux1/2
  Fcn11/1 -> Mux1/3
  Fcn12/1 -> Mux1/4
  Fcn13/1 -> Mux1/5
  Fcn14/1 -> Mux1/6
  Fcn15/1 -> Mux1/7
  Fcn16/1 -> Mux1/8
  Fcn17/1 -> Mux1/9
  Mux1/1 -> Selector/1, Selector1/1, Selector2/1  "RotationMatrix"
  Selector/1 -> Dot Product/2
  POSvector_BODY_[m]/1 -> Dot Product2/1, Dot Product1/1, Dot Product/1
  Dot Product/1 -> Mux3/1
  Selector1/1 -> Dot Product1/2
  Selector2/1 -> Dot Product2/2
  Dot Product2/1 -> Mux3/3
  Dot Product1/1 -> Mux3/2
  rot_xyz 2 rot_zyx/1 -> Fcn9/1, Fcn10/1, Fcn11/1, Fcn12/1, Fcn13/1, Fcn14/1, Fcn15/1, Fcn16/1, Fcn17/1
  Mux3/1 -> POSvector_GLOBAL_[m]/1
  angles_BODYwrtGLOB_[rad]/1 -> rot_xyz 2 rot_zyx/1

== system Demo_3D_FlexRoads_cs/Audi_A8_1/PreScan_Contact_Sensor/Vehicle Local to World/state2FullState/limit roll ==
  RPY : Inport
  Demux : Demux  Outputs=3
  Mux1 : Mux  Inputs=3
  Substitute 90 & 270 deg (and its plurals) : Subsystem
  RPYcor : Outport
  wires:
  Substitute 90 & 270 deg (and its plurals)/1(Subst Angle [rad]) -> Mux1/1
  Mux1/1 -> RPYcor/1
  RPY/1 -> Demux/1
  Demux/3 -> Mux1/3
  Demux/2 -> Mux1/2
  Demux/1 -> Substitute 90 & 270 deg (and its plurals)/1(Angle [rad])

== system Demo_3D_FlexRoads_cs/Audi_A8_1/PreScan_Contact_Sensor/Wheels Local to World/conv_RotWheelFL/RotMat2AxisAngle ==
  RotMat_Visu : Inport
  Data Type Conversion : DataTypeConversion
  Divide : Product  Inputs=*/
  Gain : Gain  Gain=2
  Mux : Mux  Inputs=3
  Mux1 : Mux  Inputs=2
  Saturation1 : Saturate  UpperLimit=3-0.001  LowerLimit=-1+0.001
  Trigonometric Function : Trigonometry
  U1 : Fcn  Expr=u[6]-u[8]
  U2 : Fcn  Expr=u[7]-u[3]
  U3 : Fcn  Expr=u[2]-u[4]
  U_Phi : Fcn  Expr=u[1]+u[5]+u[9]
  U_Phi1 : Fcn  Expr=acos((u(1)-1)/2)
  U_Phi2 : Fcn  Expr=acos((u(1)-1)/2)
  Angles_Visu : Outport
  wires:
  U_Phi2/1 -> Trigonometric Function/1
  Saturation1/1 -> U_Phi2/1
  U_Phi1/1 -> Data Type Conversion/1
  U_Phi/1 -> Saturation1/1, U_Phi1/1
  Divide/1 -> Mux1/1
  Mux1/1 -> Angles_Visu/1
  Gain/1 -> Divide/2
  Mux/1 -> Divide/1
  U3/1 -> Mux/3
  U2/1 -> Mux/2
  U1/1 -> Mux/1
  Trigonometric Function/1 -> Gain/1
  RotMat_Visu/1 -> U_Phi/1, U3/1, U2/1, U1/1
  Data Type Conversion/1 -> Mux1/2

== system Demo_3D_FlexRoads_cs/Audi_A8_1/PreScan_Contact_Sensor/Wheels Local to World/conv_RotWheelFR/RotMat2AxisAngle ==
  RotMat_Visu : Inport
  Data Type Conversion : DataTypeConversion
  Divide : Product  Inputs=*/
  Gain : Gain  Gain=2
  Mux : Mux  Inputs=3
  Mux1 : Mux  Inputs=2
  Saturation1 : Saturate  UpperLimit=3-0.001  LowerLimit=-1+0.001
  Trigonometric Function : Trigonometry
  U1 : Fcn  Expr=u[6]-u[8]
  U2 : Fcn  Expr=u[7]-u[3]
  U3 : Fcn  Expr=u[2]-u[4]
  U_Phi : Fcn  Expr=u[1]+u[5]+u[9]
  U_Phi1 : Fcn  Expr=acos((u(1)-1)/2)
  U_Phi2 : Fcn  Expr=acos((u(1)-1)/2)
  Angles_Visu : Outport
  wires:
  Data Type Conversion/1 -> Mux1/2
  RotMat_Visu/1 -> U1/1, U2/1, U3/1, U_Phi/1
  Trigonometric Function/1 -> Gain/1
  U1/1 -> Mux/1
  U2/1 -> Mux/2
  U3/1 -> Mux/3
  Mux/1 -> Divide/1
  Gain/1 -> Divide/2
  Mux1/1 -> Angles_Visu/1
  Divide/1 -> Mux1/1
  U_Phi/1 -> U_Phi1/1, Saturation1/1
  U_Phi1/1 -> Data Type Conversion/1
  Saturation1/1 -> U_Phi2/1
  U_Phi2/1 -> Trigonometric Function/1

== system Demo_3D_FlexRoads_cs/Audi_A8_1/PreScan_Contact_Sensor/Wheels Local to World/conv_RotWheelRL/RotMat2AxisAngle ==
  RotMat_Visu : Inport
  Data Type Conversion : DataTypeConversion
  Divide : Product  Inputs=*/
  Gain : Gain  Gain=2
  Mux : Mux  Inputs=3
  Mux1 : Mux  Inputs=2
  Saturation1 : Saturate  UpperLimit=3-0.001  LowerLimit=-1+0.001
  Trigonometric Function : Trigonometry
  U1 : Fcn  Expr=u[6]-u[8]
  U2 : Fcn  Expr=u[7]-u[3]
  U3 : Fcn  Expr=u[2]-u[4]
  U_Phi : Fcn  Expr=u[1]+u[5]+u[9]
  U_Phi1 : Fcn  Expr=acos((u(1)-1)/2)
  U_Phi2 : Fcn  Expr=acos((u(1)-1)/2)
  Angles_Visu : Outport
  wires:
  Data Type Conversion/1 -> Mux1/2
  RotMat_Visu/1 -> U1/1, U2/1, U3/1, U_Phi/1
  Trigonometric Function/1 -> Gain/1
  U1/1 -> Mux/1
  U2/1 -> Mux/2
  U3/1 -> Mux/3
  Mux/1 -> Divide/1
  Gain/1 -> Divide/2
  Mux1/1 -> Angles_Visu/1
  Divide/1 -> Mux1/1
  U_Phi/1 -> U_Phi1/1, Saturation1/1
  U_Phi1/1 -> Data Type Conversion/1
  Saturation1/1 -> U_Phi2/1
  U_Phi2/1 -> Trigonometric Function/1

== system Demo_3D_FlexRoads_cs/Audi_A8_1/PreScan_Contact_Sensor/Wheels Local to World/conv_RotWheelRR/RotMat2AxisAngle ==
  RotMat_Visu : Inport
  Data Type Conversion : DataTypeConversion
  Divide : Product  Inputs=*/
  Gain : Gain  Gain=2
  Mux : Mux  Inputs=3
  Mux1 : Mux  Inputs=2
  Saturation1 : Saturate  UpperLimit=3-0.001  LowerLimit=-1+0.001
  Trigonometric Function : Trigonometry
  U1 : Fcn  Expr=u[6]-u[8]
  U2 : Fcn  Expr=u[7]-u[3]
  U3 : Fcn  Expr=u[2]-u[4]
  U_Phi : Fcn  Expr=u[1]+u[5]+u[9]
  U_Phi1 : Fcn  Expr=acos((u(1)-1)/2)
  U_Phi2 : Fcn  Expr=acos((u(1)-1)/2)
  Angles_Visu : Outport
  wires:
  Data Type Conversion/1 -> Mux1/2
  RotMat_Visu/1 -> U1/1, U2/1, U3/1, U_Phi/1
  Trigonometric Function/1 -> Gain/1
  U1/1 -> Mux/1
  U2/1 -> Mux/2
  U3/1 -> Mux/3
  Mux/1 -> Divide/1
  Gain/1 -> Divide/2
  Mux1/1 -> Angles_Visu/1
  Divide/1 -> Mux1/1
  U_Phi/1 -> U_Phi1/1, Saturation1/1
  U_Phi1/1 -> Data Type Conversion/1
  Saturation1/1 -> U_Phi2/1
  U_Phi2/1 -> Trigonometric Function/1

== system Demo_3D_FlexRoads_cs/Audi_A8_1/PreScan_Contact_Sensor/Wheels Local to World/conv_TransWheelFL/pos_ini_Visu ==
  Constant : Constant  Value=x_ini_VRML
  Constant1 : Constant  Value=y_ini_VRML
  Constant2 : Constant  Value=z_ini_VRML
  Mux1 : Mux  Inputs=3
  pos_ini_Visu : Outport
  wires:
  Constant2/1 -> Mux1/3
  Constant1/1 -> Mux1/2
  Mux1/1 -> pos_ini_Visu/1
  Constant/1 -> Mux1/1
